simulink model "statespaceExSimulink0"  (R2023b)
settings: Solver=VariableStepAuto  StartTime=0.0  StopTime=10.0  RelTol=1e-3
undefined symbols (not defined in the file): A, B, C, K
settings Model: Creator=klysm  LastModifiedBy=klysm

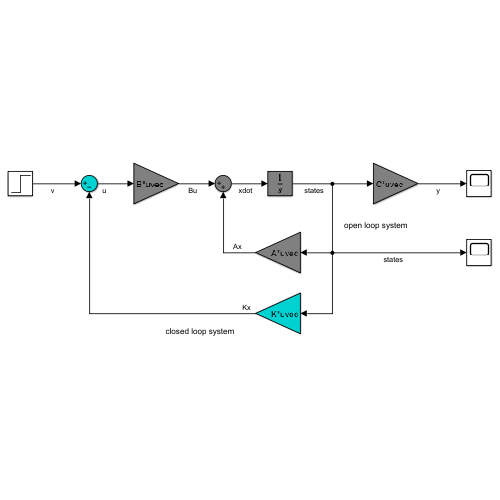
[thumbnail: Simulink's stored preview of the top-level diagram]
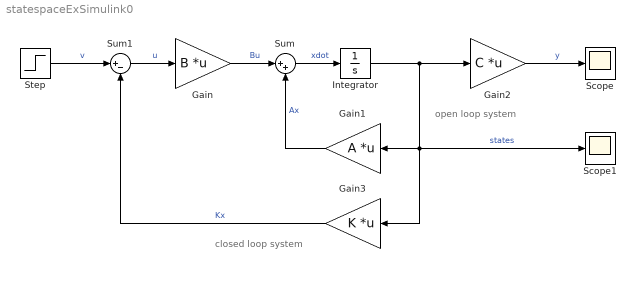
== system statespaceExSimulink0 ==
  note: open loop system
  note: closed loop system
  Gain : Gain  Gain=B  Multiplication=Matrix(K*u) (u vector)
  Gain1 : Gain  Gain=A  Multiplication=Matrix(K*u) (u vector)
  Gain2 : Gain  Gain=C  Multiplication=Matrix(K*u) (u vector)
  Gain3 : Gain  Gain=K  Multiplication=Matrix(K*u) (u vector)
  Integrator : Integrator
  Scope : Scope
  Scope1 : Scope
  Step : Step  SampleTime=0
  Sum : Sum  Inputs=|++
  Sum1 : Sum  Inputs=|+-
  wires:
  Sum/1 -> Integrator/1  "xdot"
  Gain1/1 -> Sum/2  "Ax"
  Gain/1 -> Sum/1  "Bu"
  Integrator/1 -> Gain2/1, Scope1/1, Gain1/1, Gain3/1  "states"
  Gain2/1 -> Scope/1  "y"
  Sum1/1 -> Gain/1  "u"
  Gain3/1 -> Sum1/2  "Kx"
  Step/1 -> Sum1/1  "v"
